simulink model "tb_SYSTEM"  (R2022b)
settings: Solver=FixedStepDiscrete  StartTime=0  StopTime=0.01  RelTol=1e-3
InitFcn:
  | init_SYSTEM;
values from neighbouring files (symbols this model uses):
  AD9545_INIT = bitconcat(ufi(AD9545_tmp(:,1),16,0),ufi(AD9545_tmp(:,2),8,0))    [init_SYSTEM.m]
  AXI_DDR_CONTROL = Simulink.Parameter    [init_SYSTEM.m]
  AXI_MonADC_CONTROL = Simulink.Parameter    [init_SYSTEM.m]
  AXI_MonADC_SPI_Wr = Simulink.Parameter    [init_SYSTEM.m]
  AXI_PWR_CONTROL = Simulink.Parameter    [init_SYSTEM.m]
  AXI_XAVIER_CONTROL = Simulink.Parameter    [init_SYSTEM.m]
  model_time_step = 1/80e6    (= 1.25e-08)    [init_CameraIO.m]    (also in init_SYSTEM.m)
libraries: hdlsllib x22, simulink x20
(part 1 of 2)
Description:
  | Copyright (c) 2023, Alexei Evsenin, evsenin@gmail.com
settings Model: DataTypeOverride=Off  PacingRate=0.011000  Creator=mmwoperator  LastModifiedBy=evsenin
settings SolverCC: AlgebraicLoopSolver=TrustRegion
settings DataIOCC: SaveOutput=off  DSMLogging=off  SaveTime=off
settings OptimizationCC: BlockReduction=off  ConditionallyExecuteInputs=off  DefaultParameterBehavior=Inlined  InheritOutputTypeSmallerThanSingle=on  DefaultUnderspecifiedDataType=single
settings DebuggingCC: AlgebraicLoopMsg=error  SingleTaskRateTransMsg=error  ParameterUnderflowMsg=error  ParameterPrecisionLossMsg=none  ParameterTunabilityLossMsg=error  FixptConstUnderflowMsg=warning  FixptConstOverflowMsg=warning  UnconnectedInputMsg=warning  UnconnectedOutputMsg=warning  UnconnectedLineMsg=warning  SFMachineParentedDataDiag=warning  UnderSpecifiedDimensionMsg=warning
settings HardwareCC: ProdBitPerPointer=32  ProdBitPerSizeT=32  ProdBitPerPtrDiffT=32  ProdLargestAtomicFloat=None  ProdIntDivRoundTo=Undefined  ProdEndianess=Unspecified  ProdWordSize=32  ProdHWDeviceType=ASIC/FPGA->ASIC/FPGA  TargetBitPerPointer=64  TargetBitPerSizeT=64  TargetBitPerPtrDiffT=64  TargetLongLongMode=on  TargetIntDivRoundTo=Zero  TargetEndianess=LittleEndian  TargetWordSize=64  TargetHWDeviceType=Custom Processor->MATLAB Host Computer  ProdEqTarget=off
settings ModelReferenceCC: EnableRefExpFcnMdlSchedulingChecks=on
settings SFSimCC: SimTargetLang=C++
settings RTWCC: DLArmComputeVersion=19.05

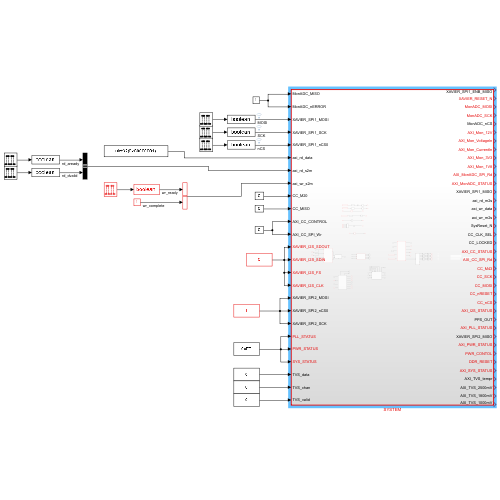
[thumbnail: Simulink's stored preview of the top-level diagram]
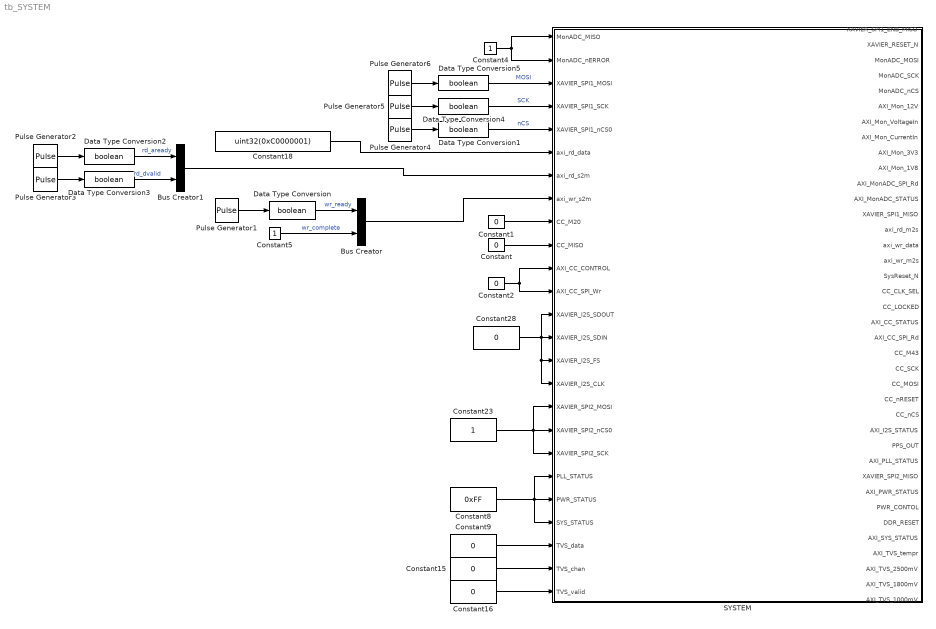
== system tb_SYSTEM ==
  Bus Creator : BusCreator  Inputs=2
  Bus Creator1 : BusCreator  Inputs=2
  Constant : Constant  Value=0  OutDataTypeStr=boolean  SampleTime=model_time_step
  Constant1 : Constant  Value=0  OutDataTypeStr=fixdt(0,3,0)  SampleTime=model_time_step
  Constant15 : Constant  Value=0  OutDataTypeStr=fixdt(0,2,0)  SampleTime=model_time_step
  Constant16 : Constant  Value=0  OutDataTypeStr=boolean  SampleTime=model_time_step
  Constant18 : Constant  Value=uint32(0xC0000001)  SampleTime=model_time_step
  Constant2 : Constant  Value=0  OutDataTypeStr=uint32  SampleTime=model_time_step
  Constant23 : Constant  OutDataTypeStr=boolean  SampleTime=model_time_step
  Constant28 : Constant  Value=0  OutDataTypeStr=boolean  SampleTime=model_time_step
  Constant4 : Constant  OutDataTypeStr=boolean  SampleTime=model_time_step
  Constant5 : Constant  OutDataTypeStr=boolean  SampleTime=model_time_step
  Constant8 : Constant  Value=0xFF  OutDataTypeStr=uint8  SampleTime=model_time_step
  Constant9 : Constant  Value=0  OutDataTypeStr=int16  SampleTime=model_time_step
  Data Type Conversion{,1..5} (6 alike) : DataTypeConversion  OutDataTypeStr=boolean  SaturateOnIntegerOverflow=off  RndMeth=Floor
  Pulse Generator1 : DiscretePulseGenerator  Period=1111  PulseWidth=555  SampleTime=model_time_step
  Pulse Generator2 : DiscretePulseGenerator  Period=1  SampleTime=model_time_step
  Pulse Generator3 : DiscretePulseGenerator  Period=1  SampleTime=model_time_step
  Pulse Generator4 : DiscretePulseGenerator  Period=194  PulseWidth=2  SampleTime=model_time_step
  Pulse Generator5 : DiscretePulseGenerator  PhaseDelay=1  SampleTime=model_time_step
  Pulse Generator6 : DiscretePulseGenerator  Period=16  PulseWidth=8  PhaseDelay=4  SampleTime=model_time_step
  SYSTEM : Subsystem  TreatAsAtomicUnit=on  SystemSampleTime=model_time_step
      settings: RTWSystemCode=Inline  PortSchema="{\"entries\":[{\"content\":{\"sides\":[{\"content\":{\"connectorIds\":[\"Out1\",\"Out2\",\"Out3\",\"Out4\",\"Out5\",\"Out6\",\"Out7\",\"Out8\",\"Out9\",\"Out10\",\"Out11\",\"Out12\",\"Out13\",\"Out14\",\"Out15\",\"Out16\",\"Out17\",\"Out18\",\"Out19\",\"Out20\",\"Out21\",\"Out22\",\"Out23\",\"Out24\",\"Out25\",\"Out26\",\"Out27\",\"Out28\",\"Out29\",\"Out30\",\"Out31\",\"Out32\",\"Out33\",\"Out34\",\"Out35\",\"Out36\",\"Out37\",\"Out38\"]},\"type\":\"ConnectorPlacement.EquallySpacedRectSide\",\"uuid\":\"5c413c8b-6069-4c75-b777-373528e2ae9d\"},{\"content\":{\"connectorIds\":[\"In1\",\"In2\",\"In3\",\"In4\",\"In5\",\"In6\",\"In7\",\"In8\",\"In9\",\"In10\",\"In11\",\"In12\",\"In13\",\"In14\",\"In15\",\"In16\",\"In17\",\"In18\",\"In19\",\"In20\",\"In21\",\"In22\",\"In23\",\"In24\",\"In25\"],\"side\":\"RIGHT\"},\"type\":\"ConnectorPlacement.EquallySpacedRectSide\",\"uuid\":\"9d073273-c858-4909-9831-9e199bb6500d\"},{\"content\":{\"connectorIds\":[],\"side\":\"TOP\"},\"type\":\"ConnectorPlacement.EquallySpacedRectSide\",\"uuid\":\"280a689a-c9d6-412c-b222-f1f9c2e69a6a\"},{\"content\":{\"connectorIds\":[],\"side\":\"BOTTOM\"},\"type\":\"ConnectorPlacement.EquallySpacedRectSide\",\"uuid\":\"933f1101-30ad-4058-a510-bd6f2b5ce475\"}]},\"type\":\"ConnectorPlacement.EquallySpacedConnector\",\"uuid\":\"a7978c0e-bed1-4344-aea7-7974b4bfe1eb\"}],\"packageUris\":[\"http://schema.mathworks.com/mf0/Connector/R2020b\"],\"version\":\"1.0\"}"
  wires:
  Constant15/1 -> SYSTEM/2(TVS_chan)
  Constant16/1 -> SYSTEM/1(TVS_valid)
  Constant9/1 -> SYSTEM/3(TVS_data)
  Constant23/1 -> SYSTEM/7(XAVIER_SPI2_SCK), SYSTEM/9(XAVIER_SPI2_MOSI), SYSTEM/8(XAVIER_SPI2_nCS0)
  Constant8/1 -> SYSTEM/6(PLL_STATUS), SYSTEM/4(SYS_STATUS), SYSTEM/5(PWR_STATUS)
  Constant28/1 -> SYSTEM/12(XAVIER_I2S_SDIN), SYSTEM/13(XAVIER_I2S_SDOUT), SYSTEM/11(XAVIER_I2S_FS), SYSTEM/10(XAVIER_I2S_CLK)
  Constant2/1 -> SYSTEM/14(AXI_CC_SPI_Wr), SYSTEM/15(AXI_CC_CONTROL)
  Constant1/1 -> SYSTEM/17(CC_M20)
  Constant/1 -> SYSTEM/16(CC_MISO)
  Pulse Generator5/1 -> Data Type Conversion4/1
  Data Type Conversion1/1 -> SYSTEM/21(XAVIER_SPI1_nCS0)  "nCS"
  Data Type Conversion4/1 -> SYSTEM/22(XAVIER_SPI1_SCK)  "SCK"
  Pulse Generator6/1 -> Data Type Conversion5/1
  Pulse Generator4/1 -> Data Type Conversion1/1
  Data Type Conversion5/1 -> SYSTEM/23(XAVIER_SPI1_MOSI)  "MOSI"
  Pulse Generator2/1 -> Data Type Conversion2/1
  Data Type Conversion3/1 -> Bus Creator1/2  "rd_dvalid"
  Data Type Conversion2/1 -> Bus Creator1/1  "rd_aready"
  Bus Creator1/1 -> SYSTEM/19(axi_rd_s2m)
  Pulse Generator3/1 -> Data Type Conversion3/1
  Constant18/1 -> SYSTEM/20(axi_rd_data)
  Pulse Generator1/1 -> Data Type Conversion/1
  Constant5/1 -> Bus Creator/2  "wr_complete"
  Data Type Conversion/1 -> Bus Creator/1  "wr_ready"
  Bus Creator/1 -> SYSTEM/18(axi_wr_s2m)
  Constant4/1 -> SYSTEM/25(MonADC_MISO), SYSTEM/24(MonADC_nERROR)

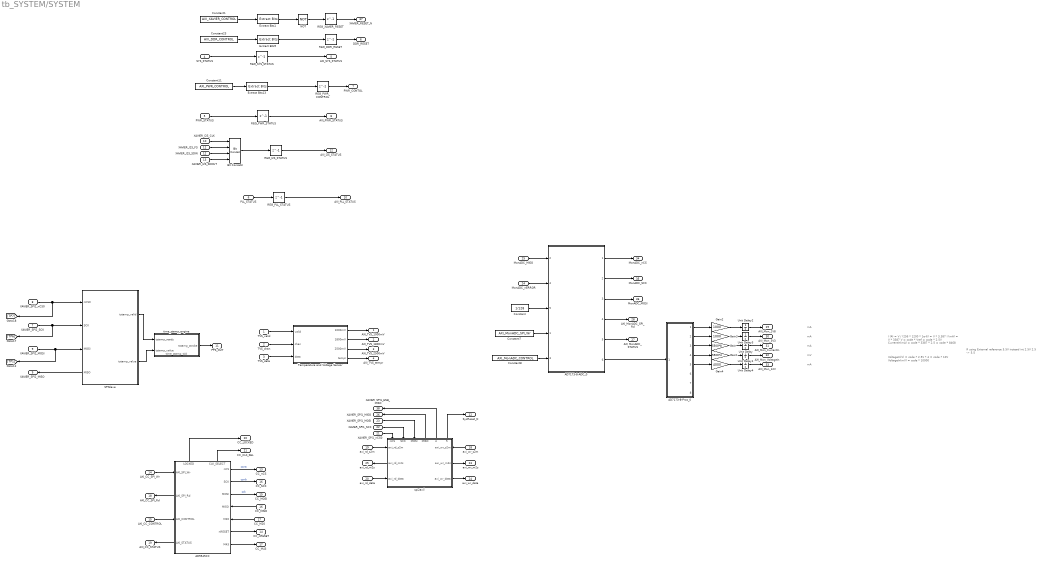
== system tb_SYSTEM/SYSTEM ==
  note: I (A) = V / (256 * 1200 * 1e-6) = V * 3.387
      | I (mA) = V * 3387
      | V = code * Vref = code * 2.5V
      | CurrentIn(mA) = code * 3387 * 2.5 = code * 8468
  note: mA
  note: If using External reference 5.5V instead int 2.5V
      | 2.5 -> 5.5
  note: VoltageIn(V) = code * 2.5V * 4 = code * 10V
      | VoltageIn(mV) = code * 10000
  note: mA
  note: mA
  note: mA
  note: mV
  TVS_valid : Inport
  TVS_chan : Inport  Port=2
  TVS_data : Inport  Port=3
  SYS_STATUS : Inport  Port=4
  PWR_STATUS : Inport  Port=5
  PLL_STATUS : Inport  Port=6
  XAVIER_SPI2_SCK : Inport  Port=7
  XAVIER_SPI2_nCS0 : Inport  Port=8
  XAVIER_SPI2_MOSI : Inport  Port=9
  XAVIER_I2S_CLK : Inport  Port=10
  XAVIER_I2S_FS : Inport  Port=11
  XAVIER_I2S_SDIN : Inport  Port=12
  XAVIER_I2S_SDOUT : Inport  Port=13
  AXI_CC_SPI_Wr : Inport  Port=14
  AXI_CC_CONTROL : Inport  Port=15
  CC_MISO : Inport  Port=16
  CC_M20 : Inport  Port=17
  axi_wr_s2m : Inport  Port=18
  axi_rd_s2m : Inport  Port=19
  axi_rd_data : Inport  Port=20
  XAVIER_SPI1_nCS0 : Inport  Port=21
  XAVIER_SPI1_SCK : Inport  Port=22
  XAVIER_SPI1_MOSI : Inport  Port=23
  MonADC_nERROR : Inport  Port=24
  MonADC_MISO : Inport  Port=25
  AD7173-8-ADC_0 : Subsystem  ReferencedSubsystem=AD7173_8_ADC
      settings: PortSchema="{\"entries\":[{\"content\":{\"sides\":[{\"content\":{\"connectorIds\":[\"In2\",\"In4\",\"In5\",\"In1\",\"In3\"]},\"type\":\"ConnectorPlacement.EquallySpacedRectSide\",\"uuid\":\"97243915-fe88-4cad-a1e4-3850b5d18a30\"},{\"content\":{\"connectorIds\":[\"Out1\",\"Out2\",\"Out3\",\"Out4\",\"Out5\",\"Out6\"],\"side\":\"RIGHT\"},\"type\":\"ConnectorPlacement.EquallySpacedRectSide\",\"uuid\":\"28d1ffa2-15a9-468b-ac8e-40a785c64adf\"},{\"content\":{\"connectorIds\":[],\"side\":\"TOP\"},\"type\":\"ConnectorPlacement.EquallySpacedRectSide\",\"uuid\":\"f19f2378-338b-455c-abf7-82f02bb25504\"},{\"content\":{\"connectorIds\":[],\"side\":\"BOTTOM\"},\"type\":\"ConnectorPlacement.EquallySpacedRectSide\",\"uuid\":\"c072e952-1c7e-4d0a-bd82-39eb15451e3b\"},{\"content\":{\"connectorIds\":[],\"side\":\"HIDDEN\"},\"type\":\"ConnectorPlacement.EquallySpacedRectSide\",\"uuid\":\"2718e8b2-cd07-4b49-a636-abcceb600b04\"}]},\"type\":\"ConnectorPlacement.EquallySpacedConnector\",\"uuid\":\"c08a06d6-e57b-40ae-a1a6-fde99cbc862e\"}],\"packageUris\":[\"http://schema.mathworks.com/mf0/Connector/R2020b\"],\"version\":\"1.0\"}"
  AD7173-8-Proc_0 : Subsystem  ReferencedSubsystem=VectorExpand
  AD9545CC : Subsystem
      settings: PortSchema="{\"entries\":[{\"content\":{\"sides\":[{\"content\":{\"connectorIds\":[\"In1\",\"Out8\",\"In2\",\"Out9\"]},\"type\":\"ConnectorPlacement.EquallySpacedRectSide\",\"uuid\":\"97243915-fe88-4cad-a1e4-3850b5d18a30\"},{\"content\":{\"connectorIds\":[\"Out1\",\"Out2\",\"Out3\",\"In3\",\"In4\",\"Out4\",\"Out5\"],\"side\":\"RIGHT\"},\"type\":\"ConnectorPlacement.EquallySpacedRectSide\",\"uuid\":\"28d1ffa2-15a9-468b-ac8e-40a785c64adf\"},{\"content\":{\"connectorIds\":[\"Out6\",\"Out7\"],\"side\":\"TOP\"},\"type\":\"ConnectorPlacement.EquallySpacedRectSide\",\"uuid\":\"f19f2378-338b-455c-abf7-82f02bb25504\"},{\"content\":{\"connectorIds\":[],\"side\":\"HIDDEN\"},\"type\":\"ConnectorPlacement.EquallySpacedRectSide\",\"uuid\":\"2718e8b2-cd07-4b49-a636-abcceb600b04\"}]},\"type\":\"ConnectorPlacement.EquallySpacedConnector\",\"uuid\":\"c08a06d6-e57b-40ae-a1a6-fde99cbc862e\"}],\"packageUris\":[\"http://schema.mathworks.com/mf0/Connector/R2020b\"],\"version\":\"1.0\"}"
  Bit Concat3 : hdlsllib/Logic and Bit Operations/Bit Concat  numInputs=4
  Constant : Constant  Value=1/128  OutDataTypeStr=fixdt(0,16,16)  SampleTime=-1
  Constant1 : Constant  Value=AXI_XAVIER_CONTROL  OutDataTypeStr=uint32  SampleTime=-1
  Constant11 : Constant  Value=AXI_PWR_CONTROL  OutDataTypeStr=uint32  SampleTime=-1
  Constant23 : Constant  Value=AXI_DDR_CONTROL  OutDataTypeStr=uint32  SampleTime=-1
  Constant7 : Constant  Value=AXI_MonADC_SPI_Wr  OutDataTypeStr=uint32  SampleTime=-1
  Constant8 : Constant  Value=AXI_MonADC_CONTROL  OutDataTypeStr=uint32  SampleTime=-1
  Extract Bits1 : simulink/Logic and Bit Operations/Extract Bits  bitsToExtract=Range of bits  numBits=8  bitIdxRange=0  outScalingMode=Treat bit field as an integer
  Extract Bits13 : simulink/Logic and Bit Operations/Extract Bits  bitsToExtract=Range of bits  numBits=8  bitIdxRange=[0 7]  outScalingMode=Treat bit field as an integer
  Extract Bits9 : simulink/Logic and Bit Operations/Extract Bits  bitsToExtract=Range of bits  numBits=8  bitIdxRange=0  outScalingMode=Treat bit field as an integer
  Gain : Gain  Gain=5500*8  OutDataTypeStr=int32
  Gain1 : Gain  Gain=5500*4  OutDataTypeStr=int32
  Gain2 : Gain  Gain=1000  OutDataTypeStr=int32
  Gain3 : Gain  Gain=1000  OutDataTypeStr=int32
  Gain4 : Gain  Gain=4000  OutDataTypeStr=int32
  NOT : Logic  Operator=NOT  IconShape=distinctive  AllPortsSameDT=off  OutDataTypeStr=boolean
  REG_DDR_RESET : Delay  DelayLength=1
  REG_I2S_STATUS : Delay  DelayLength=1
  REG_PLL_STATUS : Delay  DelayLength=1
  REG_PWR_CONTROL : Delay  DelayLength=1
  REG_PWR_STATUS : Delay  DelayLength=1
  REG_SYS_STATUS : Delay  DelayLength=1
  REG_XAVIER_RESET : Delay  DelayLength=1
  SPISlave : Subsystem
      settings: PortSchema="{\"entries\":[{\"content\":{\"sides\":[{\"content\":{\"connectorIds\":[\"In1\",\"In2\",\"In3\",\"Out3\"]},\"type\":\"ConnectorPlacement.EquallySpacedRectSide\",\"uuid\":\"988cab7b-3eb1-4078-928a-08523e84b74e\"},{\"content\":{\"connectorIds\":[\"Out1\",\"Out2\"],\"side\":\"RIGHT\"},\"type\":\"ConnectorPlacement.EquallySpacedRectSide\",\"uuid\":\"618e3cb6-b8f9-4735-8b09-0fe0436fb3aa\"},{\"content\":{\"connectorIds\":[],\"side\":\"TOP\"},\"type\":\"ConnectorPlacement.EquallySpacedRectSide\",\"uuid\":\"1ab04a62-ac70-4b76-bdb0-d54264b3534c\"}]},\"type\":\"ConnectorPlacement.EquallySpacedConnector\",\"uuid\":\"22be0427-517b-4e4b-a6b6-c604274f5841\"}],\"packageUris\":[\"http://schema.mathworks.com/mf0/Connector/R2020b\"],\"version\":\"1.0\"}"
  Temperature and Voltage Sensor : Subsystem
  Unit Delay{,1..4} (5 alike) : UnitDelay  SampleTime=-1  HasFrameUpgradeWarning=on
  spi2axil : Subsystem
      settings: PortSchema="{\"entries\":[{\"content\":{\"sides\":[{\"content\":{\"connectorIds\":[\"In1\",\"Out6\",\"In2\"]},\"type\":\"ConnectorPlacement.EquallySpacedRectSide\",\"uuid\":\"988cab7b-3eb1-4078-928a-08523e84b74e\"},{\"content\":{\"connectorIds\":[\"In6\",\"Out1\",\"Out2\"],\"side\":\"RIGHT\"},\"type\":\"ConnectorPlacement.EquallySpacedRectSide\",\"uuid\":\"618e3cb6-b8f9-4735-8b09-0fe0436fb3aa\"},{\"content\":{\"connectorIds\":[\"In3\",\"In4\",\"In5\",\"Out3\",\"Out4\",\"Out5\"],\"side\":\"TOP\"},\"type\":\"ConnectorPlacement.EquallySpacedRectSide\",\"uuid\":\"1ab04a62-ac70-4b76-bdb0-d54264b3534c\"}]},\"type\":\"ConnectorPlacement.EquallySpacedConnector\",\"uuid\":\"22be0427-517b-4e4b-a6b6-c604274f5841\"}],\"packageUris\":[\"http://schema.mathworks.com/mf0/Connector/R2020b\"],\"version\":\"1.0\"}"
  time_stamp_engine : Subsystem
      settings: PortSchema="{\"entries\":[{\"content\":{\"sides\":[{\"content\":{\"connectorIds\":[\"In1\",\"In2\"]},\"type\":\"ConnectorPlacement.EquallySpacedRectSide\",\"uuid\":\"8b602992-3bf4-437b-921b-9d5cd291ba83\"},{\"content\":{\"connectorIds\":[\"Out1\"],\"side\":\"RIGHT\"},\"type\":\"ConnectorPlacement.EquallySpacedRectSide\",\"uuid\":\"9d3def33-14b6-40e7-b01b-4f0a41ffd200\"},{\"content\":{\"connectorIds\":[],\"side\":\"TOP\"},\"type\":\"ConnectorPlacement.EquallySpacedRectSide\",\"uuid\":\"60dab4fc-fbf8-4e43-96f8-2b9b2dee4992\"},{\"content\":{\"connectorIds\":[\"Out2\"],\"side\":\"BOTTOM\"},\"type\":\"ConnectorPlacement.EquallySpacedRectSide\",\"uuid\":\"df767697-fe1c-433d-b09a-011f3dc07411\"}]},\"type\":\"ConnectorPlacement.EquallySpacedConnector\",\"uuid\":\"29f25002-e5c5-4bd7-949c-81f58631edcc\"}],\"packageUris\":[\"http://schema.mathworks.com/mf0/Connector/R2020b\"],\"version\":\"1.0\"}"
  AXI_TVS_1000mV : Outport
  AXI_TVS_1800mV : Outport  Port=2
  AXI_TVS_2500mV : Outport  Port=3
  AXI_TVS_tempr : Outport  Port=4
  AXI_SYS_STATUS : Outport  Port=5
  DDR_RESET : Outport  Port=6
  PWR_CONTOL : Outport  Port=7
  AXI_PWR_STATUS : Outport  Port=8
  XAVIER_SPI2_MISO : Outport  Port=9
  AXI_PLL_STATUS : Outport  Port=10
  PPS_OUT : Outport  Port=11
  AXI_I2S_STATUS : Outport  Port=12
  CC_nCS : Outport  Port=13
  CC_nRESET : Outport  Port=14
  CC_MOSI : Outport  Port=15
  CC_SCK : Outport  Port=16
  CC_M43 : Outport  Port=17
  AXI_CC_SPI_Rd : Outport  Port=18
  AXI_CC_STATUS : Outport  Port=19
  CC_LOCKED : Outport  Port=20
  CC_CLK_SEL : Outport  Port=21
  SysReset_N : Outport  Port=22
  axi_wr_m2s : Outport  Port=23
  axi_wr_data : Outport  Port=24
  axi_rd_m2s : Outport  Port=25
  XAVIER_SPI1_MISO : Outport  Port=26
  AXI_MonADC_STATUS : Outport  Port=27
  AXI_MonADC_SPI_Rd : Outport  Port=28
  AXI_Mon_1V8 : Outport  Port=29
  AXI_Mon_3V3 : Outport  Port=30
  AXI_Mon_CurrentIn : Outport  Port=31
  AXI_Mon_VoltageIn : Outport  Port=32
  AXI_Mon_12V : Outport  Port=33
  MonADC_nCS : Outport  Port=34
  MonADC_SCK : Outport  Port=35
  MonADC_MOSI : Outport  Port=36
  XAVIER_RESET_N : Outport  Port=37
  XAVIER_SPI1_ENB_MISO : Outport  Port=38
  wires:
  TVS_chan/1 -> Temperature and Voltage Sensor/2(chan)
  Temperature and Voltage Sensor/4(tempr) -> AXI_TVS_tempr/1
  Temperature and Voltage Sensor/3(2500mV) -> AXI_TVS_2500mV/1
  Temperature and Voltage Sensor/1(1000mV) -> AXI_TVS_1000mV/1
  TVS_valid/1 -> Temperature and Voltage Sensor/1(valid)
  Temperature and Voltage Sensor/2(1800mV) -> AXI_TVS_1800mV/1
  TVS_data/1 -> Temperature and Voltage Sensor/3(data)
  SYS_STATUS/1 -> REG_SYS_STATUS/1
  REG_SYS_STATUS/1 -> AXI_SYS_STATUS/1
  Constant23/1 -> Extract Bits9/1
  REG_DDR_RESET/1 -> DDR_RESET/1
  REG_PWR_STATUS/1 -> AXI_PWR_STATUS/1
  Extract Bits13/1 -> REG_PWR_CONTROL/1
  REG_PWR_CONTROL/1 -> PWR_CONTOL/1
  Constant11/1 -> Extract Bits13/1
  PWR_STATUS/1 -> REG_PWR_STATUS/1
  XAVIER_SPI2_MOSI/1 -> [TP1], SPISlave/3(MOSI)
  XAVIER_SPI2_nCS0/1 -> [TP7], SPISlave/1(nCS0)
  XAVIER_SPI2_SCK/1 -> [TP6], SPISlave/2(SCK)
  SPISlave/3(MISO) -> XAVIER_SPI2_MISO/1
  PLL_STATUS/1 -> REG_PLL_STATUS/1
  SPISlave/1(tstamp_valid) -> time_stamp_engine/1(tstamp_ready)
  SPISlave/2(tstamp_value) -> time_stamp_engine/2(tstamp_value)
  Extract Bits9/1 -> REG_DDR_RESET/1
  REG_PLL_STATUS/1 -> AXI_PLL_STATUS/1
  time_stamp_engine/1(tstamp_strobe) -> PPS_OUT/1
  REG_I2S_STATUS/1 -> AXI_I2S_STATUS/1
  XAVIER_I2S_CLK/1 -> Bit Concat3/1
  XAVIER_I2S_FS/1 -> Bit Concat3/2
  XAVIER_I2S_SDIN/1 -> Bit Concat3/3
  XAVIER_I2S_SDOUT/1 -> Bit Concat3/4
  Bit Concat3/1 -> REG_I2S_STATUS/1
  AD9545CC/2(SCK) -> CC_SCK/1  "csnb"
  AD9545CC/6(LOCKED) -> CC_LOCKED/1
  AD9545CC/5(M43) -> CC_M43/1
  AD9545CC/1(nCS) -> CC_nCS/1  "csna"
  AD9545CC/3(MOSI) -> CC_MOSI/1  "sck"
  AD9545CC/4(nRESET) -> CC_nRESET/1
  AD9545CC/8(AXI_SPI_Rd) -> AXI_CC_SPI_Rd/1
  AD9545CC/9(AXI_STATUS) -> AXI_CC_STATUS/1
  AD9545CC/7(CLK_SELECT) -> CC_CLK_SEL/1
  AXI_CC_SPI_Wr/1 -> AD9545CC/1(AXI_SPI_Wr)
  AXI_CC_CONTROL/1 -> AD9545CC/2(AXI_CONTROL)
  CC_MISO/1 -> AD9545CC/3(MISO)
  CC_M20/1 -> AD9545CC/4(M20)
  spi2axil/5(EXT_RST_N) -> SysReset_N/1
  spi2axil/1(axi_wr_m2s) -> axi_wr_m2s/1
  axi_wr_s2m/1 -> spi2axil/6(axi_wr_s2m)
  spi2axil/2(axi_wr_data) -> axi_wr_data/1
  axi_rd_s2m/1 -> spi2axil/1(axi_rd_s2m)
  spi2axil/6(axi_rd_m2s) -> axi_rd_m2s/1
  axi_rd_data/1 -> spi2axil/2(axi_rd_data)
  XAVIER_SPI1_nCS0/1 -> spi2axil/3(nCS)
  XAVIER_SPI1_MOSI/1 -> spi2axil/5(MOSI)
  XAVIER_SPI1_SCK/1 -> spi2axil/4(SCK)
  spi2axil/3(MISO) -> XAVIER_SPI1_MISO/1
  Constant8/1 -> AD7173-8-ADC_0/3
  AD7173-8-ADC_0/4 -> AXI_MonADC_SPI_Rd/1
  Constant7/1 -> AD7173-8-ADC_0/1
  AD7173-8-ADC_0/5 -> AXI_MonADC_STATUS/1
  Gain4/1 -> Unit Delay4/1
  Gain/1 -> Unit Delay/1
  Gain3/1 -> Unit Delay3/1
  AD7173-8-Proc_0/5 -> Gain4/1
  Gain2/1 -> Unit Delay2/1
  AD7173-8-Proc_0/2 -> Gain3/1
  AD7173-8-Proc_0/4 -> Gain1/1
  AD7173-8-Proc_0/1 -> Gain2/1
  AD7173-8-Proc_0/3 -> Gain/1
  AD7173-8-ADC_0/6 -> AD7173-8-Proc_0/1
  Gain1/1 -> Unit Delay1/1
  AD7173-8-ADC_0/3 -> MonADC_MOSI/1
  AD7173-8-ADC_0/2 -> MonADC_SCK/1
  AD7173-8-ADC_0/1 -> MonADC_nCS/1
  MonADC_MISO/1 -> AD7173-8-ADC_0/2
  MonADC_nERROR/1 -> AD7173-8-ADC_0/4
  Constant/1 -> AD7173-8-ADC_0/5
  Unit Delay/1 -> AXI_Mon_CurrentIn/1
  Unit Delay1/1 -> AXI_Mon_VoltageIn/1
  Unit Delay3/1 -> AXI_Mon_3V3/1
  Unit Delay2/1 -> AXI_Mon_1V8/1
  Unit Delay4/1 -> AXI_Mon_12V/1
  REG_XAVIER_RESET/1 -> XAVIER_RESET_N/1
  Constant1/1 -> Extract Bits1/1
  Extract Bits1/1 -> NOT/1
  NOT/1 -> REG_XAVIER_RESET/1
  spi2axil/4(ENB_MISO) -> XAVIER_SPI1_ENB_MISO/1

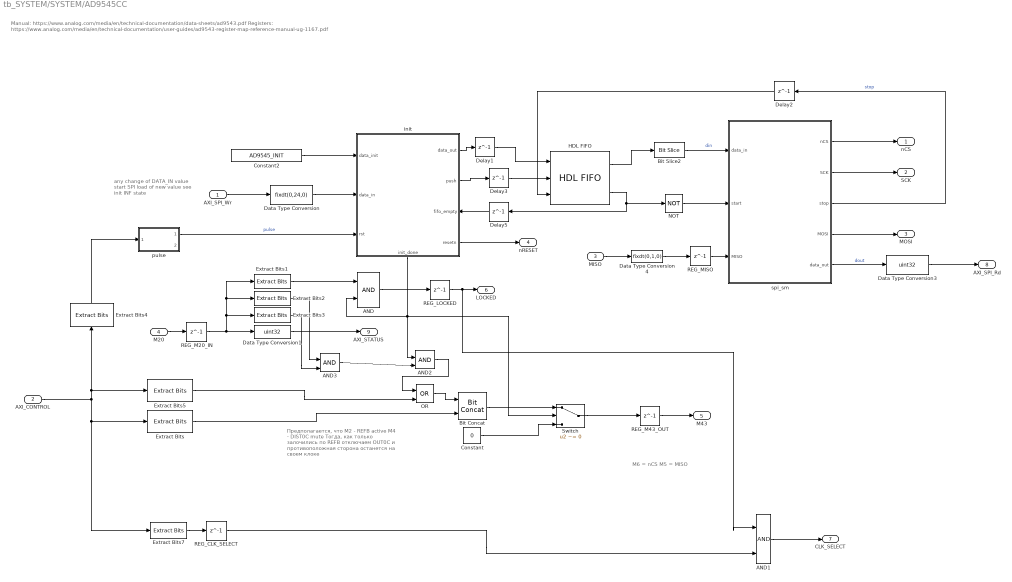
== system tb_SYSTEM/SYSTEM/AD9545CC ==
  note: Предполагается, что
      | M2 - REFB active
      | M4 - DIST0C mute
      | Тогда, как только залочились по REFB
      | отключаем OUT0C
      | и противоположная сторона останется
      | на своем клоке
  note: M6 = nCS
      | M5 = MISO
  note: Manual:
      | https://www.analog.com/media/en/technical-documentation/data-sheets/ad9543.pdf
      |
      | Registers:
      | https://www.analog.com/media/en/technical-documentation/user-guides/ad9543-register-map-reference-manual-ug-1167.pdf
  note: any change of DATA_IN value
      | start SPI load of new value
      | see init INF state
  AXI_SPI_Wr : Inport
  AXI_CONTROL : Inport  Port=2
  MISO : Inport  Port=3
  M20 : Inport  Port=4
  AND{,1..3} (4 alike) : Logic  IconShape=distinctive  AllPortsSameDT=off  OutDataTypeStr=boolean
  Bit Concat : hdlsllib/Logic and Bit Operations/Bit Concat  numInputs=2
  Bit Slice2 : hdlsllib/Logic and Bit Operations/Bit Slice  lidx=23  ridx=0
  Constant : Constant  Value=0  OutDataTypeStr=fixdt(0,2,0)  SampleTime=-1
  Constant2 : Constant  Value=AD9545_INIT  OutDataTypeStr=fixdt(0,24,0)  SampleTime=-1
  Data Type Conversion : DataTypeConversion  OutDataTypeStr=fixdt(0,24,0)  SaturateOnIntegerOverflow=off  RndMeth=Floor
  Data Type Conversion1 : DataTypeConversion  OutDataTypeStr=uint32  SaturateOnIntegerOverflow=off  RndMeth=Floor
  Data Type Conversion3 : DataTypeConversion  OutDataTypeStr=uint32  SaturateOnIntegerOverflow=off  RndMeth=Floor
  Data Type Conversion4 : DataTypeConversion  OutDataTypeStr=fixdt(0,1,0)  SaturateOnIntegerOverflow=off  RndMeth=Floor
  Delay{1..3,5} (4 alike) : Delay  DelayLength=1
  Extract Bits : simulink/Logic and Bit Operations/Extract Bits  bitsToExtract=Range of bits  numBits=8  bitIdxRange=1  outScalingMode=Treat bit field as an integer
  Extract Bits1 : simulink/Logic and Bit Operations/Extract Bits  bitsToExtract=Range of bits  numBits=8  bitIdxRange=0  outScalingMode=Treat bit field as an integer
  Extract Bits2 : simulink/Logic and Bit Operations/Extract Bits  bitsToExtract=Range of bits  numBits=8  bitIdxRange=1  outScalingMode=Treat bit field as an integer
  Extract Bits3 : simulink/Logic and Bit Operations/Extract Bits  bitsToExtract=Range of bits  numBits=8  bitIdxRange=2  outScalingMode=Treat bit field as an integer
  Extract Bits4 : simulink/Logic and Bit Operations/Extract Bits  bitsToExtract=Range of bits  numBits=8  bitIdxRange=0  outScalingMode=Treat bit field as an integer
  Extract Bits5 : simulink/Logic and Bit Operations/Extract Bits  bitsToExtract=Range of bits  numBits=8  bitIdxRange=2  outScalingMode=Treat bit field as an integer
  Extract Bits7 : simulink/Logic and Bit Operations/Extract Bits  bitsToExtract=Range of bits  numBits=8  bitIdxRange=4  outScalingMode=Treat bit field as an integer
  HDL FIFO : hdlsllib/HDL RAMs/HDL FIFO  fifo_size=64  mode=FWFT  ratio=1  push_msg=Warning  pop_msg=Warning  show_empty=on  show_full=off  show_num=off  LabelModeActiveChoice_Mode=FWFT  rst_port=off
  NOT : Logic  Operator=NOT  IconShape=distinctive  AllPortsSameDT=off  OutDataTypeStr=boolean
  OR : Logic  Operator=OR  IconShape=distinctive  AllPortsSameDT=off  OutDataTypeStr=boolean
  REG_CLK_SELECT : Delay  DelayLength=1
  REG_LOCKED : Delay  DelayLength=1
  REG_M20_IN : Delay  DelayLength=1
  REG_M43_OUT : Delay  DelayLength=1
  REG_MISO : Delay  DelayLength=1
  Switch : Switch  Criteria=u2 ~= 0  SaturateOnIntegerOverflow=off  InputSameDT=off
  init : Stateflow chart  TreatAsAtomicUnit=on
      settings: PortSchema="{\"entries\":[{\"content\":{\"sides\":[{\"content\":{\"connectorIds\":[\"In1\",\"In2\",\"In4\"]},\"type\":\"ConnectorPlacement.EquallySpacedRectSide\",\"uuid\":\"2541893e-0497-4685-a403-0c18c6ba8828\"},{\"content\":{\"connectorIds\":[\"Out2\",\"Out1\",\"In3\",\"Out3\"],\"side\":\"RIGHT\"},\"type\":\"ConnectorPlacement.EquallySpacedRectSide\",\"uuid\":\"ea7d69d9-7294-4ef3-b4a5-e03a3485fcd1\"},{\"content\":{\"connectorIds\":[],\"side\":\"TOP\"},\"type\":\"ConnectorPlacement.EquallySpacedRectSide\",\"uuid\":\"4588f9c3-6d00-4467-b78c-e50bd35827d1\"},{\"content\":{\"connectorIds\":[\"Out4\"],\"side\":\"BOTTOM\"},\"type\":\"ConnectorPlacement.EquallySpacedRectSide\",\"uuid\":\"6cf1debc-d261-40b7-9985-8c0ec2d9837a\"},{\"content\":{\"connectorIds\":[],\"side\":\"HIDDEN\"},\"type\":\"ConnectorPlacement.EquallySpacedRectSide\",\"uuid\":\"32712179-057e-4c85-bea4-acb9bd43153e\"}]},\"type\":\"ConnectorPlacement.EquallySpacedConnector\",\"uuid\":\"4c1de655-9fa7-4102-a0fe-e6132f80d46b\"}],\"packageUris\":[\"http://schema.mathworks.com/mf0/Connector/R2020b\"],\"version\":\"1.0\"}"
  pulse : Subsystem  ReferencedSubsystem=pulse
  spi_sm : Stateflow chart  TreatAsAtomicUnit=on
      settings: PortSchema="{\"entries\":[{\"content\":{\"sides\":[{\"content\":{\"connectorIds\":[\"In1\",\"In3\",\"In2\"]},\"type\":\"ConnectorPlacement.EquallySpacedRectSide\",\"uuid\":\"c873ee2d-afd2-4da8-a43b-135f6a354a0c\"},{\"content\":{\"connectorIds\":[\"Out1\",\"Out4\",\"Out5\",\"Out2\",\"Out3\"],\"side\":\"RIGHT\"},\"type\":\"ConnectorPlacement.EquallySpacedRectSide\",\"uuid\":\"424a6b82-da04-4858-9164-e360fe3abeb3\"},{\"content\":{\"connectorIds\":[],\"side\":\"TOP\"},\"type\":\"ConnectorPlacement.EquallySpacedRectSide\",\"uuid\":\"9ec86d72-b4ed-4894-a0c0-a4fac65a3c4c\"},{\"content\":{\"connectorIds\":[],\"side\":\"HIDDEN\"},\"type\":\"ConnectorPlacement.EquallySpacedRectSide\",\"uuid\":\"d113467b-580b-4249-84bc-ee2c7951f3a5\"}]},\"type\":\"ConnectorPlacement.EquallySpacedConnector\",\"uuid\":\"111a2709-fa96-4e2c-b71d-d73d8b96bd37\"}],\"packageUris\":[\"http://schema.mathworks.com/mf0/Connector/R2020b\"],\"version\":\"1.0\"}"
  nCS : Outport
  SCK : Outport  Port=2
  MOSI : Outport  Port=3
  nRESET : Outport  Port=4
  M43 : Outport  Port=5
  LOCKED : Outport  Port=6
  CLK_SELECT : Outport  Port=7
  AXI_SPI_Rd : Outport  Port=8
  AXI_STATUS : Outport  Port=9
  wires:
  Data Type Conversion4/1 -> REG_MISO/1
  Bit Slice2/1 -> spi_sm/1(data_in)  "din"
  MISO/1 -> Data Type Conversion4/1
  spi_sm/4(SCK) -> SCK/1
  spi_sm/2(MOSI) -> MOSI/1
  spi_sm/3(data_out) -> Data Type Conversion3/1  "dout"
  init/3(resetn) -> nRESET/1
  spi_sm/5(stop) -> Delay2/1  "stop"
  HDL FIFO/1 -> Bit Slice2/1
  HDL FIFO/2 -> Delay5/1, NOT/1
  NOT/1 -> spi_sm/3(start)
  Delay2/1 -> HDL FIFO/3
  init/1(push) -> Delay3/1
  init/2(data_out) -> Delay1/1
  AXI_SPI_Wr/1 -> Data Type Conversion/1
  Data Type Conversion/1 -> init/2(data_in)
  Data Type Conversion3/1 -> AXI_SPI_Rd/1
  spi_sm/1(nCS) -> nCS/1
  Constant2/1 -> init/1(data_init)
  Data Type Conversion1/1 -> AXI_STATUS/1
  M20/1 -> REG_M20_IN/1
  Switch/1 -> REG_M43_OUT/1
  Constant/1 -> Switch/3
  Extract Bits1/1 -> AND/1
  AND/1 -> REG_LOCKED/1
  REG_MISO/1 -> spi_sm/2(MISO)
  init/4(init_done) -> AND2/1, AND/2, Switch/2
  REG_M20_IN/1 -> Extract Bits3/1, Extract Bits2/1, Extract Bits1/1, Data Type Conversion1/1
  REG_M43_OUT/1 -> M43/1
  Delay1/1 -> HDL FIFO/1
  Delay3/1 -> HDL FIFO/2
  Delay5/1 -> init/3(fifo_empty)
  Extract Bits4/1 -> pulse/1
  pulse/1 -> init/4(rst)  "pulse"
  Extract Bits7/1 -> REG_CLK_SELECT/1
  AND1/1 -> CLK_SELECT/1
  REG_CLK_SELECT/1 -> AND1/2
  REG_LOCKED/1 -> AND1/1, LOCKED/1
  AXI_CONTROL/1 -> Extract Bits7/1, Extract Bits/1, Extract Bits5/1, Extract Bits4/1
  Extract Bits5/1 -> OR/2
  OR/1 -> Bit Concat/1
  Extract Bits/1 -> Bit Concat/2
  Bit Concat/1 -> Switch/1
  AND2/1 -> OR/1
  Extract Bits3/1 -> AND3/2
  Extract Bits2/1 -> AND3/1
  AND3/1 -> AND2/2

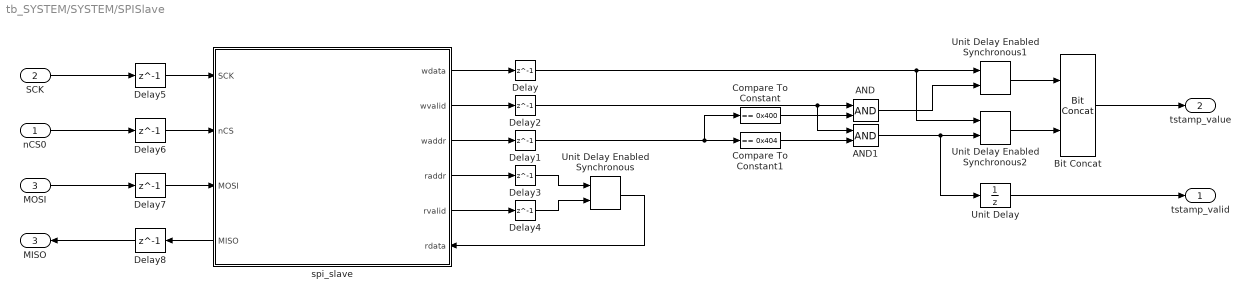
== system tb_SYSTEM/SYSTEM/SPISlave ==
  nCS0 : Inport
  SCK : Inport  Port=2
  MOSI : Inport  Port=3
  AND : Logic  IconShape=distinctive  AllPortsSameDT=off  OutDataTypeStr=boolean
  AND1 : Logic  IconShape=distinctive  AllPortsSameDT=off  OutDataTypeStr=boolean
  Bit Concat : hdlsllib/Logic and Bit Operations/Bit Concat  numInputs=2
  Compare To Constant : simulink/Logic and Bit Operations/Compare To Constant  relop===  const=0x400  OutDataTypeStr=boolean
  Compare To Constant1 : simulink/Logic and Bit Operations/Compare To Constant  relop===  const=0x404  OutDataTypeStr=boolean
  Delay{,1..8} (9 alike) : Delay  DelayLength=1
  Unit Delay : UnitDelay  SampleTime=-1  HasFrameUpgradeWarning=on
  Unit Delay Enabled Synchronous : hdlsllib/Discrete/Unit Delay Enabled Synchronous  InitialCondition=0.0  SampleTime=-1
  Unit Delay Enabled Synchronous1 : hdlsllib/Discrete/Unit Delay Enabled Synchronous  InitialCondition=0.0  SampleTime=-1
  Unit Delay Enabled Synchronous2 : hdlsllib/Discrete/Unit Delay Enabled Synchronous  InitialCondition=0.0  SampleTime=-1
  spi_slave : Stateflow chart  TreatAsAtomicUnit=on
      settings: PortSchema="{\"entries\":[{\"content\":{\"sides\":[{\"content\":{\"connectorIds\":[\"In3\",\"In1\",\"In2\",\"Out1\"]},\"type\":\"ConnectorPlacement.EquallySpacedRectSide\",\"uuid\":\"33f55eae-aa90-449d-a4d7-65fdb1be0732\"},{\"content\":{\"connectorIds\":[\"Out4\",\"Out2\",\"Out5\",\"Out6\",\"Out3\",\"In4\"],\"side\":\"RIGHT\"},\"type\":\"ConnectorPlacement.EquallySpacedRectSide\",\"uuid\":\"2d53bb47-0acb-43e3-a00b-45e7b46e7b56\"},{\"content\":{\"connectorIds\":[],\"side\":\"TOP\"},\"type\":\"ConnectorPlacement.EquallySpacedRectSide\",\"uuid\":\"c7779534-9ad2-40b7-883b-84bc3a9df088\"},{\"content\":{\"connectorIds\":[],\"side\":\"BOTTOM\"},\"type\":\"ConnectorPlacement.EquallySpacedRectSide\",\"uuid\":\"c2bbdc7a-55cc-49d8-a1e1-7534a51ba169\"}]},\"type\":\"ConnectorPlacement.EquallySpacedConnector\",\"uuid\":\"e189e830-5b57-4c09-9fb8-eb3899d9ec4e\"}],\"packageUris\":[\"http://schema.mathworks.com/mf0/Connector/R2020b\"],\"version\":\"1.0\"}"
  tstamp_valid : Outport
  tstamp_value : Outport  Port=2
  MISO : Outport  Port=3
  wires:
  spi_slave/1(MISO) -> Delay8/1
  spi_slave/2(wvalid) -> Delay2/1
  spi_slave/3(rvalid) -> Delay4/1
  spi_slave/4(wdata) -> Delay/1
  spi_slave/5(waddr) -> Delay1/1
  spi_slave/6(raddr) -> Delay3/1
  Unit Delay Enabled Synchronous/1 -> spi_slave/4(rdata)
  SCK/1 -> Delay5/1
  nCS0/1 -> Delay6/1
  MOSI/1 -> Delay7/1
  Delay4/1 -> Unit Delay Enabled Synchronous/2
  Delay3/1 -> Unit Delay Enabled Synchronous/1
  Delay1/1 -> Compare To Constant/1, Compare To Constant1/1
  Compare To Constant/1 -> AND/2
  Compare To Constant1/1 -> AND1/2
  Delay/1 -> Unit Delay Enabled Synchronous2/1, Unit Delay Enabled Synchronous1/1
  Delay2/1 -> AND/1, AND1/1
  AND/1 -> Unit Delay Enabled Synchronous1/2
  AND1/1 -> Unit Delay/1, Unit Delay Enabled Synchronous2/2
  Unit Delay Enabled Synchronous1/1 -> Bit Concat/1
  Unit Delay Enabled Synchronous2/1 -> Bit Concat/2
  Bit Concat/1 -> tstamp_value/1
  Unit Delay/1 -> tstamp_valid/1
  Delay5/1 -> spi_slave/3(SCK)
  Delay6/1 -> spi_slave/1(nCS)
  Delay7/1 -> spi_slave/2(MOSI)
  Delay8/1 -> MISO/1

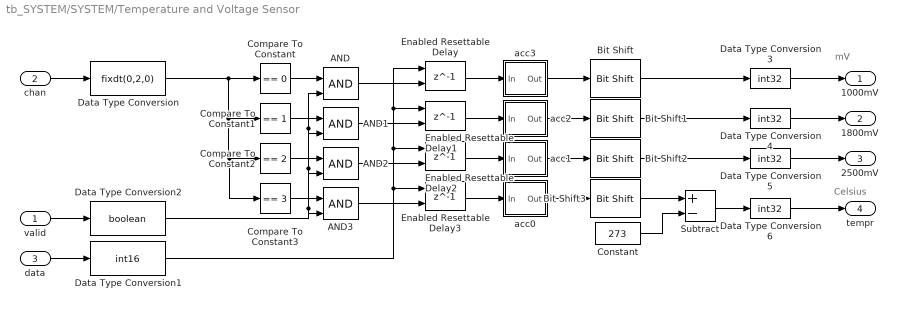
== system tb_SYSTEM/SYSTEM/Temperature and Voltage Sensor ==
  note: Celsius
  note: mV
  valid : Inport
  chan : Inport  Port=2
  data : Inport  Port=3
  AND{,1..3} (4 alike) : Logic  IconShape=distinctive  AllPortsSameDT=off  OutDataTypeStr=boolean
  Bit Shift : hdlsllib/Logic and Bit Operations/Bit Shift  mode=Shift Right Arithmetic  N=3
  Bit Shift1 : hdlsllib/Logic and Bit Operations/Bit Shift  mode=Shift Right Arithmetic  N=3
  Bit Shift2 : hdlsllib/Logic and Bit Operations/Bit Shift  mode=Shift Right Arithmetic  N=3
  Bit Shift3 : hdlsllib/Logic and Bit Operations/Bit Shift  mode=Shift Right Arithmetic  N=4
  Compare To Constant : simulink/Logic and Bit Operations/Compare To Constant  relop===  const=0  OutDataTypeStr=boolean
  Compare To Constant1 : simulink/Logic and Bit Operations/Compare To Constant  relop===  const=1  OutDataTypeStr=boolean
  Compare To Constant2 : simulink/Logic and Bit Operations/Compare To Constant  relop===  const=2  OutDataTypeStr=boolean
  Compare To Constant3 : simulink/Logic and Bit Operations/Compare To Constant  relop===  const=3  OutDataTypeStr=boolean
  Constant : Constant  Value=273  OutDataTypeStr=int16  SampleTime=-1
  Data Type Conversion : DataTypeConversion  OutDataTypeStr=fixdt(0,2,0)  SaturateOnIntegerOverflow=off  RndMeth=Floor
  Data Type Conversion1 : DataTypeConversion  OutDataTypeStr=int16  SaturateOnIntegerOverflow=off  RndMeth=Floor
  Data Type Conversion2 : DataTypeConversion  OutDataTypeStr=boolean  SaturateOnIntegerOverflow=off  RndMeth=Floor
  Data Type Conversion{3..6} (4 alike) : DataTypeConversion  OutDataTypeStr=int32  SaturateOnIntegerOverflow=off  RndMeth=Floor
  Enabled Resettable Delay{,1..3} (4 alike) : Delay  DelayLength=1  ShowEnablePort=on
      settings: InputPortMap=u0,e6
  Subtract : Sum  Inputs=+-  AccumDataTypeStr=int16  OutDataTypeStr=int16  SaturateOnIntegerOverflow=on
  acc0 : Subsystem
  acc1 : Subsystem
  acc2 : Subsystem
  acc3 : Subsystem
  1000mV : Outport
  1800mV : Outport  Port=2
  2500mV : Outport  Port=3
  tempr : Outport  Port=4
  wires:
  Data Type Conversion1/1 -> Enabled Resettable Delay/1, Enabled Resettable Delay1/1, Enabled Resettable Delay2/1, Enabled Resettable Delay3/1
  Enabled Resettable Delay/1 -> acc3/1(In)
  Enabled Resettable Delay1/1 -> acc2/1(In)
  Enabled Resettable Delay2/1 -> acc1/1(In)
  Data Type Conversion/1 -> Compare To Constant3/1, Compare To Constant2/1, Compare To Constant1/1, Compare To Constant/1
  Compare To Constant/1 -> AND/1
  Compare To Constant1/1 -> AND1/1
  Compare To Constant2/1 -> AND2/1
  Compare To Constant3/1 -> AND3/1
  valid/1 -> Data Type Conversion2/1
  AND/1 -> Enabled Resettable Delay/2
  AND1/1 -> Enabled Resettable Delay1/2
  AND2/1 -> Enabled Resettable Delay2/2
  AND3/1 -> Enabled Resettable Delay3/2
  chan/1 -> Data Type Conversion/1
  data/1 -> Data Type Conversion1/1
  Data Type Conversion2/1 -> AND/2, AND1/2, AND2/2, AND3/2
  Bit Shift/1 -> Data Type Conversion3/1
  Bit Shift1/1 -> Data Type Conversion4/1
  Bit Shift2/1 -> Data Type Conversion5/1
  Enabled Resettable Delay3/1 -> acc0/1(In)
  Constant/1 -> Subtract/2
  Subtract/1 -> Data Type Conversion6/1
  Data Type Conversion3/1 -> 1000mV/1
  Data Type Conversion4/1 -> 1800mV/1
  Data Type Conversion5/1 -> 2500mV/1
  Data Type Conversion6/1 -> tempr/1
  Bit Shift3/1 -> Subtract/1
  acc0/1(Out) -> Bit Shift3/1
  acc1/1(Out) -> Bit Shift2/1
  acc2/1(Out) -> Bit Shift1/1
  acc3/1(Out) -> Bit Shift/1

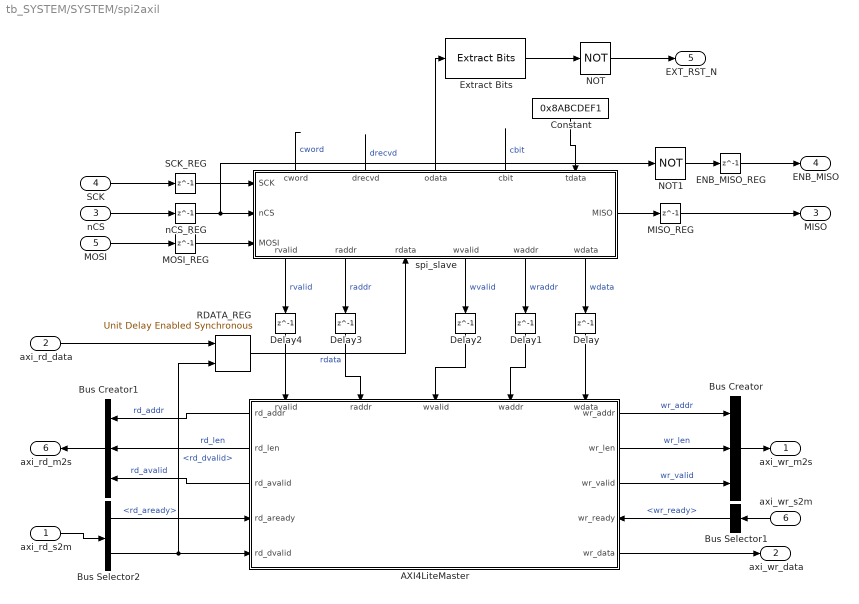
== system tb_SYSTEM/SYSTEM/spi2axil ==
  axi_rd_s2m : Inport
  axi_rd_data : Inport  Port=2
  nCS : Inport  Port=3
  SCK : Inport  Port=4
  MOSI : Inport  Port=5
  axi_wr_s2m : Inport  Port=6
  AXI4LiteMaster : Stateflow chart  TreatAsAtomicUnit=on
      settings: PortSchema="{\"entries\":[{\"content\":{\"sides\":[{\"content\":{\"connectorIds\":[\"Out4\",\"Out6\",\"Out5\",\"In3\",\"Out7\"]},\"type\":\"ConnectorPlacement.EquallySpacedRectSide\",\"uuid\":\"0b53d01b-361c-4469-afee-067f03397172\"},{\"content\":{\"connectorIds\":[\"Out1\",\"Out2\",\"Out3\",\"In1\",\"In2\"],\"side\":\"RIGHT\"},\"type\":\"ConnectorPlacement.EquallySpacedRectSide\",\"uuid\":\"9fe9e429-0d8f-4cf0-ac39-63f6e01cf4a8\"},{\"content\":{\"connectorIds\":[\"In5\",\"In6\",\"In4\",\"In8\",\"In7\"],\"side\":\"TOP\"},\"type\":\"ConnectorPlacement.EquallySpacedRectSide\",\"uuid\":\"53fd090c-8adf-4eeb-8317-8ba007d9316c\"},{\"content\":{\"connectorIds\":[],\"side\":\"BOTTOM\"},\"type\":\"ConnectorPlacement.EquallySpacedRectSide\",\"uuid\":\"119d770b-1fa7-416f-bbea-0a85945bb0a3\"}]},\"type\":\"ConnectorPlacement.EquallySpacedConnector\",\"uuid\":\"ee94014b-83df-4ad3-882a-bd43022e49b2\"}],\"packageUris\":[\"http://schema.mathworks.com/mf0/Connector/R2020b\"],\"version\":\"1.0\"}"
  Bus Creator : BusCreator  Inputs=3
  Bus Creator1 : BusCreator  Inputs=3
  Bus Selector1 : BusSelector  OutputSignals=wr_ready
  Bus Selector2 : BusSelector  OutputSignals=rd_aready,rd_dvalid
  Constant : Constant  Value=0x8ABCDEF1  OutDataTypeStr=uint32  SampleTime=-1
  Delay{,1..4} (5 alike) : Delay  DelayLength=1
  ENB_MISO_REG : Delay  DelayLength=1
  Extract Bits : simulink/Logic and Bit Operations/Extract Bits  bitsToExtract=Range of bits  numBits=8  bitIdxRange=31  outScalingMode=Preserve fixed-point scaling
  MISO_REG : Delay  DelayLength=1
  MOSI_REG : Delay  DelayLength=1
  NOT : Logic  Operator=NOT  IconShape=distinctive  AllPortsSameDT=off  OutDataTypeStr=boolean
  NOT1 : Logic  Operator=NOT  IconShape=distinctive  AllPortsSameDT=off  OutDataTypeStr=boolean
  RDATA_REG : hdlsllib/Discrete/Unit Delay Enabled Synchronous  InitialCondition=0.0  SampleTime=-1
  SCK_REG : Delay  DelayLength=1
  nCS_REG : Delay  DelayLength=1
  spi_slave : Stateflow chart  TreatAsAtomicUnit=on
      settings: PortSchema="{\"entries\":[{\"content\":{\"sides\":[{\"content\":{\"connectorIds\":[\"In3\",\"In1\",\"In2\"]},\"type\":\"ConnectorPlacement.EquallySpacedRectSide\",\"uuid\":\"33f55eae-aa90-449d-a4d7-65fdb1be0732\"},{\"content\":{\"connectorIds\":[\"Out1\"],\"side\":\"RIGHT\"},\"type\":\"ConnectorPlacement.EquallySpacedRectSide\",\"uuid\":\"2d53bb47-0acb-43e3-a00b-45e7b46e7b56\"},{\"content\":{\"connectorIds\":[\"Out8\",\"Out9\",\"Out10\",\"Out7\",\"In5\"],\"side\":\"TOP\"},\"type\":\"ConnectorPlacement.EquallySpacedRectSide\",\"uuid\":\"c7779534-9ad2-40b7-883b-84bc3a9df088\"},{\"content\":{\"connectorIds\":[\"Out3\",\"Out6\",\"In4\",\"Out2\",\"Out5\",\"Out4\"],\"side\":\"BOTTOM\"},\"type\":\"ConnectorPlacement.EquallySpacedRectSide\",\"uuid\":\"c2bbdc7a-55cc-49d8-a1e1-7534a51ba169\"}]},\"type\":\"ConnectorPlacement.EquallySpacedConnector\",\"uuid\":\"e189e830-5b57-4c09-9fb8-eb3899d9ec4e\"}],\"packageUris\":[\"http://schema.mathworks.com/mf0/Connector/R2020b\"],\"version\":\"1.0\"}"
  axi_wr_m2s : Outport
  axi_wr_data : Outport  Port=2
  MISO : Outport  Port=3
  ENB_MISO : Outport  Port=4
  EXT_RST_N : Outport  Port=5
  axi_rd_m2s : Outport  Port=6
  wires:
  AXI4LiteMaster/5(wr_valid) -> Bus Creator/3  "wr_valid"
  AXI4LiteMaster/4(wr_addr) -> Bus Creator/1  "wr_addr"
  AXI4LiteMaster/6(wr_len) -> Bus Creator/2  "wr_len"
  Bus Selector1/1 -> AXI4LiteMaster/3(wr_ready)  "<wr_ready>"
  Bus Selector2/1 -> AXI4LiteMaster/1(rd_aready)  "<rd_aready>"
  AXI4LiteMaster/3(rd_avalid) -> Bus Creator1/3  "rd_avalid"
  AXI4LiteMaster/1(rd_addr) -> Bus Creator1/1  "rd_addr"
  Bus Selector2/2 -> RDATA_REG/2, AXI4LiteMaster/2(rd_dvalid)  "<rd_dvalid>"
  AXI4LiteMaster/2(rd_len) -> Bus Creator1/2  "rd_len"
  spi_slave/2(wvalid) -> Delay2/1  "wvalid"
  spi_slave/3(rvalid) -> Delay4/1  "rvalid"
  spi_slave/4(wdata) -> Delay/1  "wdata"
  spi_slave/5(waddr) -> Delay1/1  "wraddr"
  spi_slave/6(raddr) -> Delay3/1  "raddr"
  RDATA_REG/1 -> spi_slave/4(rdata)  "rdata"
  SCK/1 -> SCK_REG/1
  nCS/1 -> nCS_REG/1
  MOSI/1 -> MOSI_REG/1
  Bus Creator/1 -> axi_wr_m2s/1
  axi_wr_s2m/1 -> Bus Selector1/1
  Bus Creator1/1 -> axi_rd_m2s/1
  axi_rd_s2m/1 -> Bus Selector2/1
  axi_rd_data/1 -> RDATA_REG/1
  AXI4LiteMaster/7(wr_data) -> axi_wr_data/1
  Delay/1 -> AXI4LiteMaster/5(wdata)
  Delay1/1 -> AXI4LiteMaster/6(waddr)
  Delay2/1 -> AXI4LiteMaster/4(wvalid)
  Delay3/1 -> AXI4LiteMaster/8(raddr)
  Delay4/1 -> AXI4LiteMaster/7(rvalid)
  spi_slave/1(MISO) -> MISO_REG/1
  spi_slave/8(cword) -> ?  "cword"
  spi_slave/9(drecvd) -> ?  "drecvd"
  spi_slave/7(cbit) -> ?  "cbit"
  Constant/1 -> spi_slave/5(tdata)
  SCK_REG/1 -> spi_slave/3(SCK)
  nCS_REG/1 -> NOT1/1, spi_slave/1(nCS)
  MOSI_REG/1 -> spi_slave/2(MOSI)
  MISO_REG/1 -> MISO/1
  spi_slave/10(odata) -> Extract Bits/1
  Extract Bits/1 -> NOT/1
  NOT/1 -> EXT_RST_N/1
  NOT1/1 -> ENB_MISO_REG/1
  ENB_MISO_REG/1 -> ENB_MISO/1

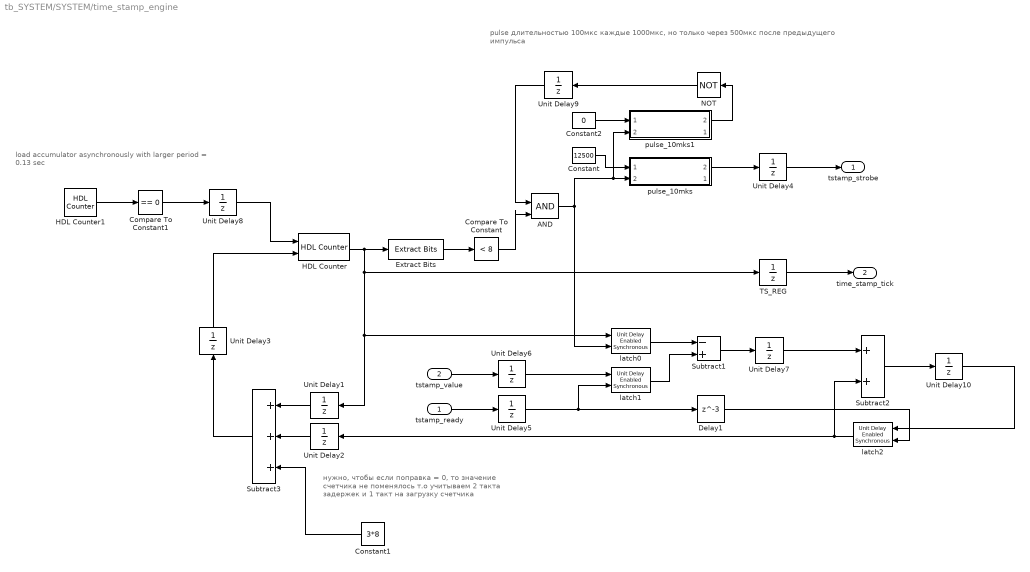
== system tb_SYSTEM/SYSTEM/time_stamp_engine ==
  note: load accumulator asynchronously
      | with larger period = 0.13 sec
  note: pulse длительностью 100мкс каждые 1000мкс,
      | но только через 500мкс после предыдущего импульса
  note: нужно, чтобы если поправка = 0,
      | то значение счетчика не поменялось
      | т.о учитываем 2 такта задержек и
      | 1 такт на загрузку счетчика
  tstamp_ready : Inport
  tstamp_value : Inport  Port=2
  AND : Logic  IconShape=distinctive  AllPortsSameDT=off  OutDataTypeStr=boolean
  Compare To Constant : simulink/Logic and Bit Operations/Compare To Constant  relop=<  const=8  OutDataTypeStr=boolean
  Compare To Constant1 : simulink/Logic and Bit Operations/Compare To Constant  relop===  const=0  OutDataTypeStr=boolean
  Constant : Constant  Value=12500  OutDataTypeStr=uint16  SampleTime=-1
  Constant1 : Constant  Value=3*8  OutDataTypeStr=uint64  SampleTime=-1
  Constant2 : Constant  Value=0  OutDataTypeStr=uint16  SampleTime=-1
  Delay1 : Delay  DelayLength=3
  Extract Bits : simulink/Logic and Bit Operations/Extract Bits  bitsToExtract=Range of bits  numBits=8  bitIdxRange=[0 20]  outScalingMode=Treat bit field as an integer
  HDL Counter : hdlsllib/Sources/HDL Counter  CountType=Free running  CountInit=0  CountStep=8  CountMax=25  CountFromType=Initial value  CountFrom=0  CountResetPort=off  CountLoadPort=on  CountEnbPort=off  CountDirPort=off  CountHitOutputPort=off  CountDataType=Unsigned  CountWordLen=64  CountFracLen=0  CountSampTime=-1
  HDL Counter1 : hdlsllib/Sources/HDL Counter  CountType=Free running  CountInit=1  CountStep=1  CountMax=25  CountFromType=Initial value  CountFrom=1  CountResetPort=off  CountLoadPort=off  CountEnbPort=off  CountDirPort=off  CountHitOutputPort=off  CountDataType=Unsigned  CountWordLen=24  CountFracLen=0  CountSampTime=-1
  NOT : Logic  Operator=NOT  IconShape=distinctive  AllPortsSameDT=off  OutDataTypeStr=boolean
  Subtract1 : Sum  Inputs=-+  AccumDataTypeStr=int64  OutDataTypeStr=int64
  Subtract2 : Sum  AccumDataTypeStr=int64  OutDataTypeStr=int64  SaturateOnIntegerOverflow=on
  Subtract3 : Sum  Inputs=+++  AccumDataTypeStr=int64  OutDataTypeStr=uint64  SaturateOnIntegerOverflow=on
  TS_REG : UnitDelay  SampleTime=-1  HasFrameUpgradeWarning=on
  Unit Delay{1..10} (10 alike) : UnitDelay  SampleTime=-1  HasFrameUpgradeWarning=on
  latch0 : hdlsllib/Discrete/Unit Delay Enabled Synchronous  InitialCondition=0.0  SampleTime=-1
  latch1 : hdlsllib/Discrete/Unit Delay Enabled Synchronous  InitialCondition=0.0  SampleTime=-1
  latch2 : hdlsllib/Discrete/Unit Delay Enabled Synchronous  InitialCondition=0.0  SampleTime=-1
  pulse_10mks : Subsystem  ReferencedSubsystem=pulse_extender
      settings: PortSchema="{\"entries\":[{\"content\":{\"sides\":[{\"content\":{\"connectorIds\":[\"In1\",\"In2\"]},\"type\":\"ConnectorPlacement.EquallySpacedRectSide\",\"uuid\":\"2d1d75a4-fb93-48b3-bd41-3be487260f65\"},{\"content\":{\"connectorIds\":[\"Out2\",\"Out1\"],\"side\":\"RIGHT\"},\"type\":\"ConnectorPlacement.EquallySpacedRectSide\",\"uuid\":\"e5f5e67c-9039-4e96-9cf2-9d15788519b6\"},{\"content\":{\"connectorIds\":[],\"side\":\"TOP\"},\"type\":\"ConnectorPlacement.EquallySpacedRectSide\",\"uuid\":\"7fce8485-b5db-4345-96df-b27b7baf6cb0\"},{\"content\":{\"connectorIds\":[],\"side\":\"BOTTOM\"},\"type\":\"ConnectorPlacement.EquallySpacedRectSide\",\"uuid\":\"79653104-294b-48ae-8c63-7c0ee909730a\"}]},\"type\":\"ConnectorPlacement.EquallySpacedConnector\",\"uuid\":\"7969cdf2-3f06-4483-a132-3b9d881856ed\"}],\"packageUris\":[\"http://schema.mathworks.com/mf0/Connector/R2020b\"],\"version\":\"1.0\"}"
  pulse_10mks1 : Subsystem  ReferencedSubsystem=pulse_extender
      settings: PortSchema="{\"entries\":[{\"content\":{\"sides\":[{\"content\":{\"connectorIds\":[\"In1\",\"In2\"]},\"type\":\"ConnectorPlacement.EquallySpacedRectSide\",\"uuid\":\"2d1d75a4-fb93-48b3-bd41-3be487260f65\"},{\"content\":{\"connectorIds\":[\"Out2\",\"Out1\"],\"side\":\"RIGHT\"},\"type\":\"ConnectorPlacement.EquallySpacedRectSide\",\"uuid\":\"e5f5e67c-9039-4e96-9cf2-9d15788519b6\"},{\"content\":{\"connectorIds\":[],\"side\":\"TOP\"},\"type\":\"ConnectorPlacement.EquallySpacedRectSide\",\"uuid\":\"7fce8485-b5db-4345-96df-b27b7baf6cb0\"},{\"content\":{\"connectorIds\":[],\"side\":\"BOTTOM\"},\"type\":\"ConnectorPlacement.EquallySpacedRectSide\",\"uuid\":\"79653104-294b-48ae-8c63-7c0ee909730a\"}]},\"type\":\"ConnectorPlacement.EquallySpacedConnector\",\"uuid\":\"7969cdf2-3f06-4483-a132-3b9d881856ed\"}],\"packageUris\":[\"http://schema.mathworks.com/mf0/Connector/R2020b\"],\"version\":\"1.0\"}"
  tstamp_strobe : Outport
  time_stamp_tick : Outport  Port=2
  wires:
  HDL Counter/1 -> latch0/1, Unit Delay1/1, TS_REG/1, Extract Bits/1
  Extract Bits/1 -> Compare To Constant/1
  tstamp_ready/1 -> Unit Delay5/1
  Subtract2/1 -> Unit Delay10/1
  TS_REG/1 -> time_stamp_tick/1
  pulse_10mks/2 -> Unit Delay4/1
  Constant/1 -> pulse_10mks/1
  tstamp_value/1 -> Unit Delay6/1
  latch0/1 -> Subtract1/1
  latch1/1 -> Subtract1/2
  Subtract1/1 -> Unit Delay7/1
  Unit Delay7/1 -> Subtract2/1
  AND/1 -> pulse_10mks1/2, pulse_10mks/2, latch0/2
  Unit Delay4/1 -> tstamp_strobe/1
  Unit Delay5/1 -> latch1/2, Delay1/1
  Unit Delay6/1 -> latch1/1
  Compare To Constant/1 -> AND/2
  NOT/1 -> Unit Delay9/1
  Unit Delay9/1 -> AND/1
  pulse_10mks1/2 -> NOT/1
  Constant2/1 -> pulse_10mks1/1
  latch2/1 -> Unit Delay2/1, Subtract2/2
  Delay1/1 -> latch2/2
  Unit Delay1/1 -> Subtract3/1
  Unit Delay2/1 -> Subtract3/2
  Unit Delay3/1 -> HDL Counter/2
  Subtract3/1 -> Unit Delay3/1
  Unit Delay8/1 -> HDL Counter/1
  Constant1/1 -> Subtract3/3
  HDL Counter1/1 -> Compare To Constant1/1
  Compare To Constant1/1 -> Unit Delay8/1
  Unit Delay10/1 -> latch2/1

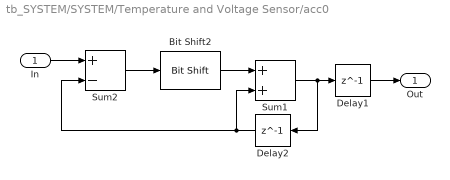
== system tb_SYSTEM/SYSTEM/Temperature and Voltage Sensor/acc0 ==
  In : Inport
  Bit Shift2 : hdlsllib/Logic and Bit Operations/Bit Shift  mode=Shift Right Arithmetic  N=6
  Delay1 : Delay  DelayLength=1
  Delay2 : Delay  DelayLength=1
  Sum1 : Sum  AccumDataTypeStr=int16  OutDataTypeStr=Inherit: Same as accumulator  SaturateOnIntegerOverflow=on
  Sum2 : Sum  Inputs=+-  AccumDataTypeStr=int16  OutDataTypeStr=Inherit: Same as accumulator  SaturateOnIntegerOverflow=on
  Out : Outport
  wires:
  Sum1/1 -> Delay1/1, Delay2/1
  In/1 -> Sum2/1
  Sum2/1 -> Bit Shift2/1
  Delay2/1 -> Sum2/2, Sum1/2
  Bit Shift2/1 -> Sum1/1
  Delay1/1 -> Out/1

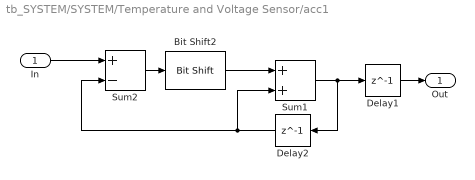
== system tb_SYSTEM/SYSTEM/Temperature and Voltage Sensor/acc1 ==
  In : Inport
  Bit Shift2 : hdlsllib/Logic and Bit Operations/Bit Shift  mode=Shift Right Arithmetic  N=6
  Delay1 : Delay  DelayLength=1
  Delay2 : Delay  DelayLength=1
  Sum1 : Sum  AccumDataTypeStr=int16  OutDataTypeStr=Inherit: Same as accumulator  SaturateOnIntegerOverflow=on
  Sum2 : Sum  Inputs=+-  AccumDataTypeStr=int16  OutDataTypeStr=Inherit: Same as accumulator  SaturateOnIntegerOverflow=on
  Out : Outport
  wires:
  Sum1/1 -> Delay1/1, Delay2/1
  In/1 -> Sum2/1
  Sum2/1 -> Bit Shift2/1
  Delay2/1 -> Sum1/2, Sum2/2
  Bit Shift2/1 -> Sum1/1
  Delay1/1 -> Out/1

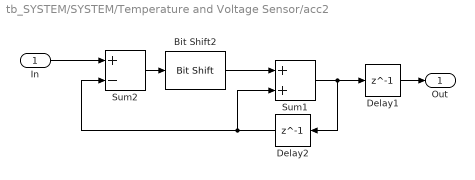
== system tb_SYSTEM/SYSTEM/Temperature and Voltage Sensor/acc2 ==
  In : Inport
  Bit Shift2 : hdlsllib/Logic and Bit Operations/Bit Shift  mode=Shift Right Arithmetic  N=6
  Delay1 : Delay  DelayLength=1
  Delay2 : Delay  DelayLength=1
  Sum1 : Sum  AccumDataTypeStr=int16  OutDataTypeStr=Inherit: Same as accumulator  SaturateOnIntegerOverflow=on
  Sum2 : Sum  Inputs=+-  AccumDataTypeStr=int16  OutDataTypeStr=Inherit: Same as accumulator  SaturateOnIntegerOverflow=on
  Out : Outport
  wires:
  Sum1/1 -> Delay1/1, Delay2/1
  In/1 -> Sum2/1
  Sum2/1 -> Bit Shift2/1
  Delay2/1 -> Sum1/2, Sum2/2
  Bit Shift2/1 -> Sum1/1
  Delay1/1 -> Out/1

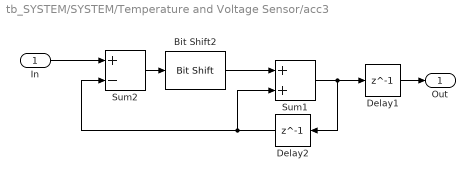
== system tb_SYSTEM/SYSTEM/Temperature and Voltage Sensor/acc3 ==
  In : Inport
  Bit Shift2 : hdlsllib/Logic and Bit Operations/Bit Shift  mode=Shift Right Arithmetic  N=6
  Delay1 : Delay  DelayLength=1
  Delay2 : Delay  DelayLength=1
  Sum1 : Sum  AccumDataTypeStr=int16  OutDataTypeStr=Inherit: Same as accumulator  SaturateOnIntegerOverflow=on
  Sum2 : Sum  Inputs=+-  AccumDataTypeStr=int16  OutDataTypeStr=Inherit: Same as accumulator  SaturateOnIntegerOverflow=on
  Out : Outport
  wires:
  Sum1/1 -> Delay1/1, Delay2/1
  In/1 -> Sum2/1
  Sum2/1 -> Bit Shift2/1
  Delay2/1 -> Sum1/2, Sum2/2
  Bit Shift2/1 -> Sum1/1
  Delay1/1 -> Out/1

== stateflow chart tb_SYSTEM/SYSTEM/spi2axil/spi_slave ==
  settings: executeAtInitialization=1
  state BIT_LATCH
    cbit = cbit + 1;
    %
    drecvd = bitset(drecvd, cbit, MOSI);
    oper = bitand(drecvd,uint32(0x3));
    %
    if cbit == nbit
    if oper == 0 & cword == 0
    waddr = bitand(drecvd,0xFFFFFFFC);
    next_data_write = true;
    elseif oper == 3  & cword == 0
    rvalid = true;
    raddr = bitand(drecvd,0xFFFFFFFC);
    next_data_read = true;
    elseif oper == 2  & cword == 0
    next_data_test = true;
    odata = drecvd;
    elseif next_data_write
    wvalid = true;
    wdata = drecvd;
    if cword > 1
    waddr = waddr + 4;
    end
    end
    cword = cword + 1;
    end
    % first 1M axi space without dummy word
    if cbit == 20 & oper == 1 & cword == 0
    rvalid = true;
    raddr = bitand(drecvd,0x000FFFFC);
    next_data_read = true;
    end
    %
    if cbit == nbit
    cbit = 0;
    end
    %
    if next_data_read & ...
    cword > 0 & ...
    bitget(rdata,cbit+1) == 1
    MISO = true;
    elseif next_data_test & ...
    bitget(tdata,cbit+1) == 1
    MISO = true;
    else
    MISO = false;
    end
  state CLK_HIGH_WAIT
    wvalid = false;
    rvalid = false;
  state RESET
    MISO = false;
    cbit = uint8(0);
    cword = uint8(0);
    drecvd = uint32(0);
    next_data_write = false;
    next_data_read = false;
    next_data_test = false;
    wvalid = false;
    waddr = uint32(0);
    wdata = uint32(0);
    rvalid = false;
    raddr = uint32(0);
    oper = uint32(0);
    odata = uint32(0);
  state IDLE
    cbit = 0;
    wvalid = false;
    rvalid = false;
    next_data_write = false;
    next_data_read = false;
    next_data_test = false;
    cword = 0;
    MISO = false;
    oper = 0;
    drecvd = 0;
  state CLK_LOW_WAIT
    wvalid = false;
    rvalid = false;
  BIT_LATCH -> IDLE [order 1] : [nCS]
  (default) -> RESET
  CLK_HIGH_WAIT -> BIT_LATCH [order 2] : [SCK]
  CLK_HIGH_WAIT -> IDLE [order 1] : [nCS]
  BIT_LATCH -> CLK_HIGH_WAIT [order 2] : [~SCK]
  RESET -> IDLE
  IDLE -> CLK_HIGH_WAIT : [~nCS]
  CLK_LOW_WAIT -> CLK_HIGH_WAIT [order 2] : [~SCK]
  CLK_LOW_WAIT -> IDLE [order 1] : [nCS]
  BIT_LATCH -> CLK_LOW_WAIT [order 3]
  data: nCS input boolean; MOSI input boolean; MISO output boolean; SCK input boolean; wvalid output boolean; rvalid output boolean; wdata output uint32; waddr output uint32; raddr output uint32; rdata input uint32; nbit constant uint8 =32; next_data_write local boolean; cbit output uint8; cword output uint8; drecvd output uint32; oper local uint32; next_data_read local boolean; next_data_test local boolean; tdata input uint32; odata output uint32
